simulink model "afm_z_dist_sin_est"  (R2018a)
settings: Solver=VariableStepAuto  StartTime=0.0  StopTime=trun  RelTol=1e-3
undefined symbols (not defined in the file): Cdd, ens1, ens2, K, Lz, M, Nbar, sys_obs, Ts, x0_obs
libraries: cstblocks x1
settings Model: Creator=arnold  LastModifiedBy=arnold

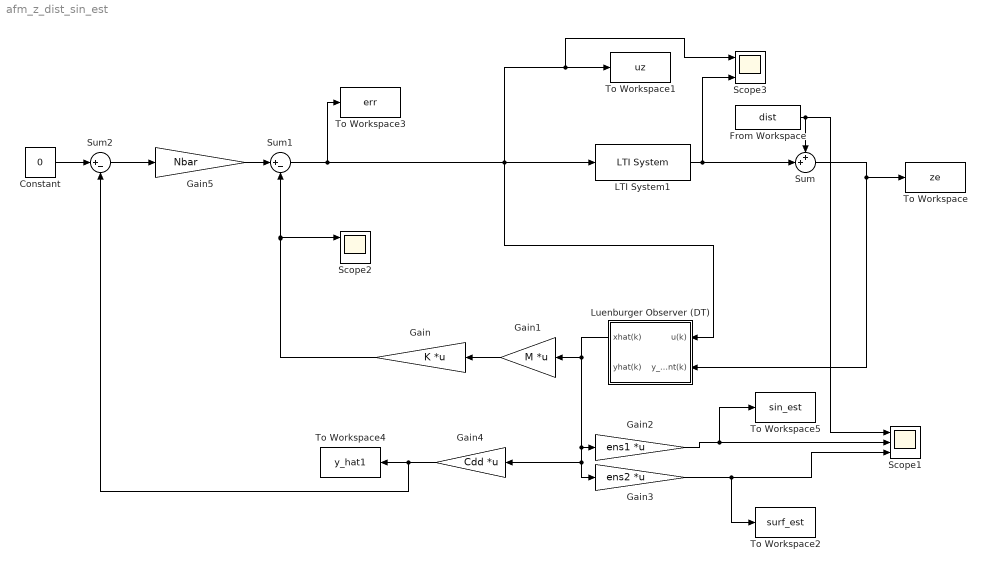
== system afm_z_dist_sin_est ==
  Constant : Constant  Value=0
  From Workspace : FromWorkspace  VariableName=dist  SampleTime=0
  Gain : Gain  Gain=K  Multiplication=Matrix(K*u)
  Gain1 : Gain  Gain=M  Multiplication=Matrix(K*u) (u vector)
  Gain2 : Gain  Gain=ens1  Multiplication=Matrix(K*u) (u vector)
  Gain3 : Gain  Gain=ens2  Multiplication=Matrix(K*u) (u vector)
  Gain4 : Gain  Gain=Cdd  Multiplication=Matrix(K*u)
  Gain5 : Gain  Gain=Nbar
  LTI System1 : cstblocks/LTI System  sys=G  IC=[]
  Luenburger Observer (DT) : Subsystem  AncestorBlock=customLibFcns/Luenburger Observer (DT)
  Scope1 : Scope  NumInputPorts=3
  Scope2 : Scope  NumInputPorts=3
  Scope3 : Scope  NumInputPorts=3
  Sum : Sum  Inputs=++|
  Sum1 : Sum  Inputs=|+-
  Sum2 : Sum  Inputs=|+-
  To Workspace : ToWorkspace  VariableName=ze  SaveFormat=Timeseries  SampleTime=-1
  To Workspace1 : ToWorkspace  VariableName=uz  SaveFormat=Timeseries  SampleTime=-1
  To Workspace2 : ToWorkspace  VariableName=surf_est  SaveFormat=Timeseries  SampleTime=-1
  To Workspace3 : ToWorkspace  VariableName=err  SaveFormat=Timeseries  SampleTime=-1
  To Workspace4 : ToWorkspace  VariableName=y_hat1  SaveFormat=Timeseries  SampleTime=-1
      settings: Save2DSignal=2-D array (concatenate along first dimension)
  To Workspace5 : ToWorkspace  VariableName=sin_est  SaveFormat=Timeseries  SampleTime=-1
  wires:
  From Workspace/1 -> Sum/1, Scope1/1
  LTI System1/1 -> Scope3/3, Sum/2
  Sum/1 -> Luenburger Observer (DT)/2(y_plant(k)), To Workspace/1
  Luenburger Observer (DT)/1(xhat(k)) -> Gain1/1, Gain4/1, Gain3/1, Gain2/1
  Gain2/1 -> To Workspace5/1, Scope1/2
  Gain1/1 -> Gain/1
  Gain4/1 -> Sum2/2, To Workspace4/1
  Gain/1 -> Sum1/2, Scope2/1
  Gain3/1 -> To Workspace2/1, Scope1/3
  Sum2/1 -> Gain5/1
  Gain5/1 -> Sum1/1
  Constant/1 -> Sum2/1
  Sum1/1 -> To Workspace3/1, LTI System1/1, Scope3/1, To Workspace1/1, Luenburger Observer (DT)/1(u(k))

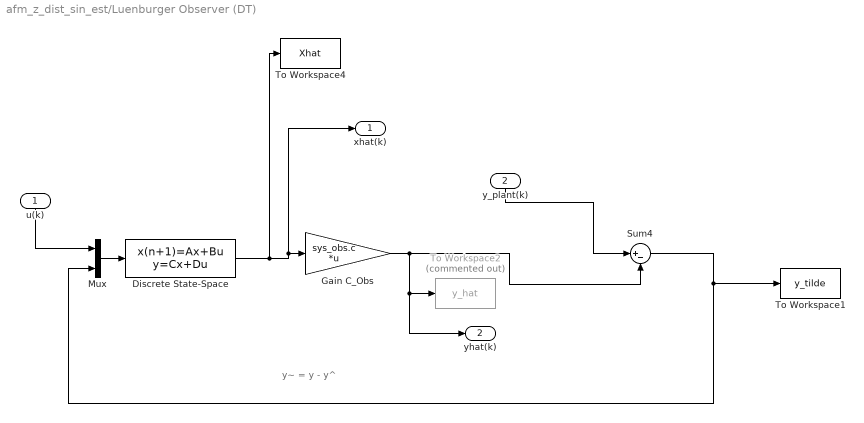
== system afm_z_dist_sin_est/Luenburger Observer (DT) ==
  note: y~ = y - y^
  u(k) : Inport
  y_plant(k) : Inport  Port=2
  Discrete State-Space : DiscreteStateSpace  A=sys_obs.a  B=[sys_obs.b, Lz]  C=eye(length(sys_obs.b))  D=zeros(length(sys_obs.b), 2)  InitialCondition=x0_obs  SampleTime=Ts
  Gain C_Obs : Gain  Gain=sys_obs.c  Multiplication=Matrix(K*u)
  Mux : Mux  Inputs=2
  Sum4 : Sum  Inputs=|+-
  To Workspace1 : ToWorkspace  VariableName=y_tilde  SaveFormat=Timeseries  SampleTime=-1
      settings: Save2DSignal=2-D array (concatenate along first dimension)
  To Workspace2 : ToWorkspace  Commented=on  VariableName=y_hat  SaveFormat=Timeseries  SampleTime=-1
      settings: Save2DSignal=2-D array (concatenate along first dimension)
  To Workspace4 : ToWorkspace  VariableName=Xhat  SaveFormat=Timeseries  SampleTime=-1
      settings: Save2DSignal=2-D array (concatenate along first dimension)
  xhat(k) : Outport
  yhat(k) : Outport  Port=2
  wires:
  Mux/1 -> Discrete State-Space/1
  Gain C_Obs/1 -> yhat(k)/1, To Workspace2/1, Sum4/2
  y_plant(k)/1 -> Sum4/1
  Discrete State-Space/1 -> xhat(k)/1, Gain C_Obs/1, To Workspace4/1
  u(k)/1 -> Mux/1
  Sum4/1 -> To Workspace1/1, Mux/2
